simulink model "Logic"  (R2025b)
settings: configuration reference "MCConfiguration" (kept outside this file)
undefined symbols (not defined in the file or in its folder): Ts_ControlFOC, Ts_Supervision
settings Model: DataDictionary=embeddedBoard_common.sldd  Creator=rpumpo  LastModifiedBy=rpumpo
settings ConfigSetRef: SourceName=MCConfiguration

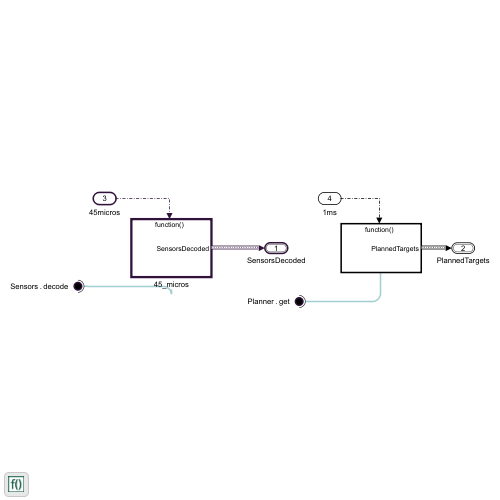
[thumbnail: Simulink's stored preview of the top-level diagram]
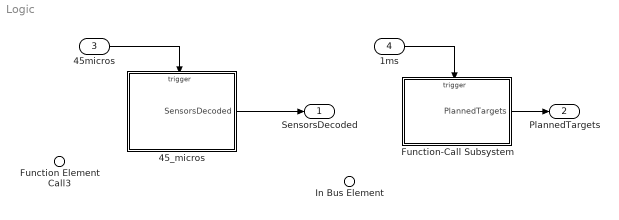
== system Logic ==
  Function Element Call3 : Inport  AllowServiceAccess=on  PortName=Sensors  Element=decode
  In Bus Element : Inport  Port=2  AllowServiceAccess=on  PortName=Planner  Element=get
  45micros : Inport  Port=3  SampleTime=Ts_ControlFOC  OutputFunctionCall=on
  1ms : Inport  Port=4  SampleTime=Ts_Supervision  OutputFunctionCall=on
  45_micros : Subsystem
  Function-Call Subsystem : Subsystem  TreatAsAtomicUnit=on
  SensorsDecoded : Outport  OutDataTypeStr=Bus: SensorsData  BusOutputAsStruct=on
  PlannedTargets : Outport  Port=2  OutDataTypeStr=Bus: Targets  BusOutputAsStruct=on
  wires:
  1ms/1 -> Function-Call Subsystem/Trigger
  45_micros/1(SensorsDecoded) -> SensorsDecoded/1
  Function-Call Subsystem/1(PlannedTargets) -> PlannedTargets/1
  45micros/1 -> 45_micros/Trigger

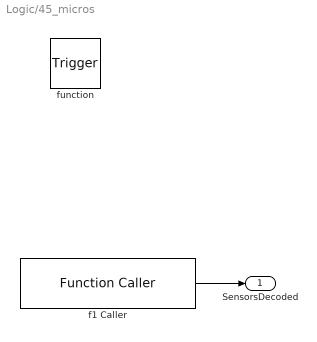
== system Logic/45_micros ==
  function : TriggerPort  TriggerType=function-call  VariantControl=(inherit)
  f1 Caller : FunctionCaller  FunctionPrototype=Sensors = Sensors.decode()  InputArgumentSpecifications=<Enter example>  OutputArgumentSpecifications=SensorsData
  SensorsDecoded : Outport  OutDataTypeStr=Bus: SensorsData
  wires:
  f1 Caller/1 -> SensorsDecoded/1

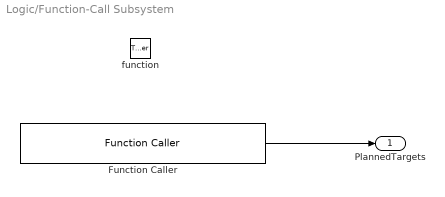
== system Logic/Function-Call Subsystem ==
  function : TriggerPort  TriggerType=function-call  VariantControl=(inherit)
  Function Caller : FunctionCaller  FunctionPrototype=PlannedTargets = Planner.get()  InputArgumentSpecifications=<Enter example>  OutputArgumentSpecifications=Targets
  PlannedTargets : Outport  OutDataTypeStr=Bus: Targets
  wires:
  Function Caller/1 -> PlannedTargets/1
